simulink model "contractTest"  (R2017a)
settings: Solver=FixedStepDiscrete  StartTime=0.0  StopTime=10.0  FixedStep=1  RelTol=1e-3
model workspace (MAT data in the model file):
  Var = 0
undefined symbols (not defined in the file or in its folder): contractAfterSimulation, contractBeforeSimulation
undefined symbols (not defined in the file): ContractAssumeBlock, ContractBlock, ContractEnsureBlock, ContractGuaranteeBlock, ContractModeBlock, ContractRequireBlock, ContractValidatorBlock
settings Model: Creator=mudat  LastModifiedBy=mahgoubyahia

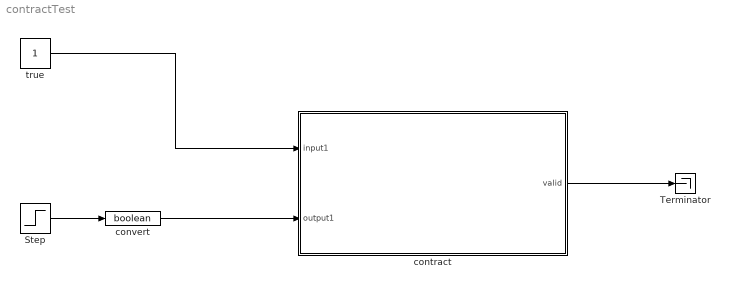
== system contractTest ==
  Step : Step  SampleTime=0
  Terminator : Terminator
  contract : Subsystem  AncestorBlock=Kind/contract  mask{ContractBlockType=ContractBlock}
      mask DialogControl DescTextVar Prompt: Contract block
      mask Display: text(0.5, 0.5, '{\bf\fontsize{20}Contract}', 'hor', 'center', 'texmode','on');
  convert : DataTypeConversion  OutDataTypeStr=boolean
  true : Constant  OutDataTypeStr=boolean
  wires:
  Step/1 -> convert/1
  convert/1 -> contract/2(output1)
  contract/1(valid) -> Terminator/1
  true/1 -> contract/1(input1)

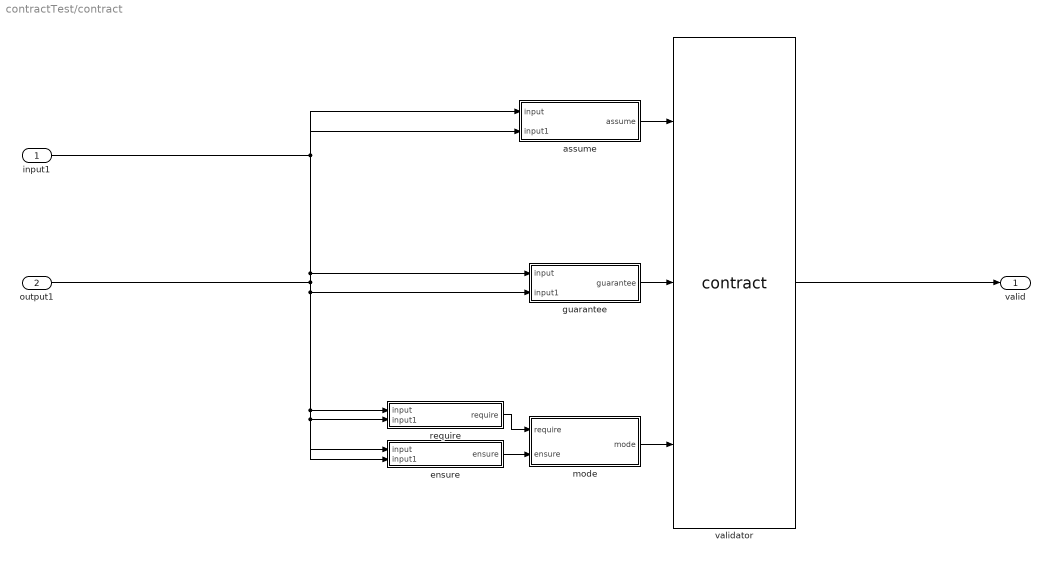
== system contractTest/contract ==
  input1 : Inport
  output1 : Inport  Port=2
  assume : Subsystem  AncestorBlock=Kind/assume  mask{ContractBlockType=ContractAssumeBlock}
      mask DialogControl DescTextVar Prompt: Assume block
  ensure : Subsystem  AncestorBlock=Kind/ensure  mask{ContractBlockType=ContractEnsureBlock}
      mask DialogControl DescTextVar Prompt: Ensure block
  guarantee : Subsystem  AncestorBlock=Kind/guarantee  mask{ContractBlockType=ContractGuaranteeBlock}
      mask DialogControl DescTextVar Prompt: Guarantee block
  mode : Subsystem  AncestorBlock=Kind/mode  mask{ContractBlockType=ContractModeBlock}
      mask DialogControl DescTextVar Prompt: Mode block
  require : Subsystem  AncestorBlock=Kind/require  mask{ContractBlockType=ContractRequireBlock}
      mask DialogControl DescTextVar Prompt: Require block
  validator : M-S-Function  InitFcn=contractBeforeSimulation();  StopFcn=contractAfterSimulation();  FunctionName=contract  mask{assumePorts=1, guaranteePorts=1, modePorts=1, ContractBlockType=ContractValidatorBlock}
      mask prompts: assumePorts "Assume ports     :"; guaranteePorts "Guarantee ports :"; modePorts "Mode ports        :"
      mask init:
      | set_param(gcb,'LinkStatus','none');
      mask Callback modePorts: contract_callback('inputs_callback',gcb)
      mask Display:
      | port_label('input',1,'assume')
      | port_label('input',2,'guarantee')
      | port_label('input',3,'mode')
      | port_label('output',1,'valid')
  valid : Outport
  wires:
  validator/1 -> valid/1
  input1/1 -> require/1(input), ensure/1(input), guarantee/1(input), assume/1(input)
  output1/1 -> require/2(input1), ensure/2(input1), guarantee/2(input1), assume/2(input1)
  assume/1(assume) -> validator/1
  guarantee/1(guarantee) -> validator/2
  mode/1(mode) -> validator/3
  require/1(require) -> mode/1(require)
  ensure/1(ensure) -> mode/2(ensure)

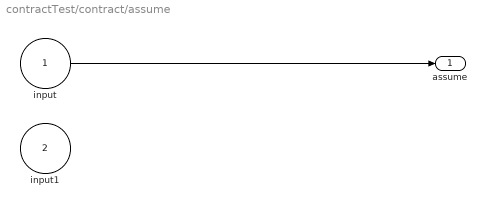
== system contractTest/contract/assume ==
  input : Inport
  input1 : Inport  Port=2
  assume : Outport  OutDataTypeStr=boolean
  wires:
  input/1 -> assume/1

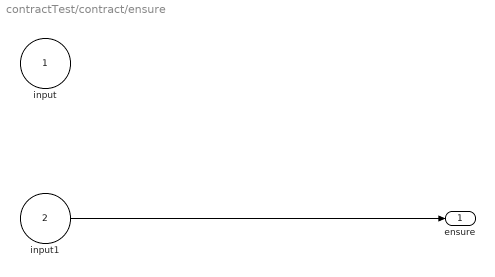
== system contractTest/contract/ensure ==
  input : Inport
  input1 : Inport  Port=2
  ensure : Outport  OutDataTypeStr=boolean
  wires:
  input1/1 -> ensure/1

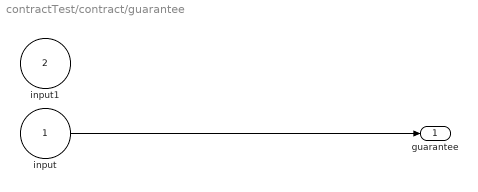
== system contractTest/contract/guarantee ==
  input : Inport
  input1 : Inport  Port=2
  guarantee : Outport  OutDataTypeStr=boolean
  wires:
  input/1 -> guarantee/1

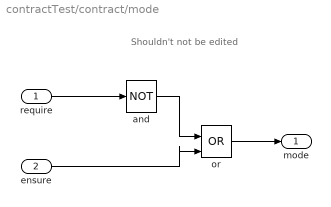
== system contractTest/contract/mode ==
  note: Shouldn't not be edited
  require : Inport  OutDataTypeStr=boolean
  ensure : Inport  Port=2  OutDataTypeStr=boolean
  and : Logic  Operator=NOT  IconShape=distinctive  AllPortsSameDT=off  OutDataTypeStr=boolean
  or : Logic  Operator=OR  IconShape=distinctive  AllPortsSameDT=off  OutDataTypeStr=boolean
  mode : Outport
  wires:
  require/1 -> and/1
  ensure/1 -> or/2
  and/1 -> or/1
  or/1 -> mode/1

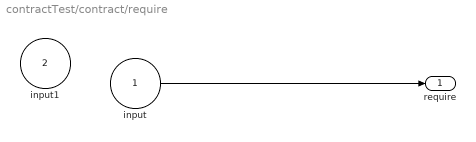
== system contractTest/contract/require ==
  input : Inport
  input1 : Inport  Port=2
  require : Outport  OutDataTypeStr=boolean
  wires:
  input/1 -> require/1
